simulink model "N_WS"  (R2024b)
settings: Solver=VariableStepAuto  StartTime=0.0  StopTime=10.0  RelTol=1e-3
values from neighbouring files (symbols this model uses):
  Ga = 0.095    [P1.m]
  Gf = 1    [P1.m]
  Gs = 1    [P1.m]
libraries: cstblocks x2
settings Model: Creator=lucap  LastModifiedBy=lucap

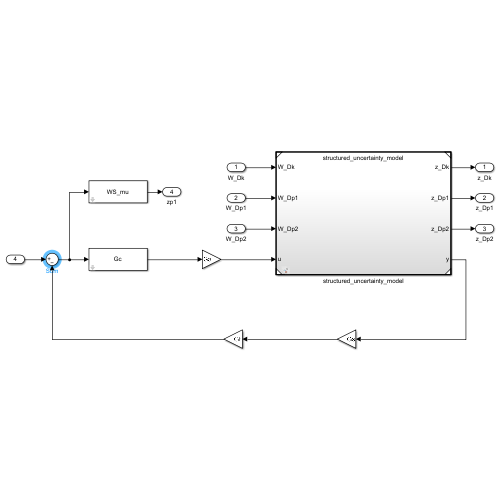
[thumbnail: Simulink's stored preview of the top-level diagram]
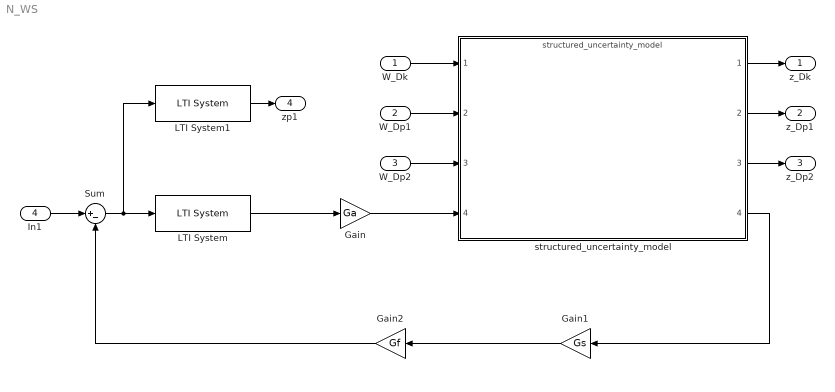
== system N_WS ==
  W_Dk : Inport
  W_Dp1 : Inport  Port=2
  W_Dp2 : Inport  Port=3
  In1 : Inport  Port=4
  Gain : Gain  Gain=Ga
  Gain1 : Gain  Gain=Gs
  Gain2 : Gain  Gain=Gf
  LTI System : cstblocks/LTI System  sys=Gc  IC=[]  PadeOrder=0
  LTI System1 : cstblocks/LTI System  sys=WS_mu  IC=[]  PadeOrder=0
  Sum : Sum  Inputs=|+-
  structured_uncertainty_model : ModelReference  ModelNameDialog=structured_uncertainty_model.slx  SimulationMode=Normal  ModelReferenceVersion=1.3
  z_Dk : Outport
  z_Dp1 : Outport  Port=2
  z_Dp2 : Outport  Port=3
  zp1 : Outport  Port=4
  wires:
  LTI System/1 -> Gain/1
  Gain/1 -> structured_uncertainty_model/4
  Sum/1 -> LTI System1/1, LTI System/1
  Gain1/1 -> Gain2/1
  Gain2/1 -> Sum/2
  structured_uncertainty_model/4 -> Gain1/1
  W_Dk/1 -> structured_uncertainty_model/1
  W_Dp1/1 -> structured_uncertainty_model/2
  W_Dp2/1 -> structured_uncertainty_model/3
  structured_uncertainty_model/1 -> z_Dk/1
  structured_uncertainty_model/2 -> z_Dp1/1
  structured_uncertainty_model/3 -> z_Dp2/1
  LTI System1/1 -> zp1/1
  In1/1 -> Sum/1
